simulink model "P2_2"  (R2024b)
settings: Solver=VariableStepAuto  StartTime=0.0  StopTime=0.1  MaxStep=T*samples  RelTol=1e-3
values from neighbouring files (symbols this model uses):
  C = 200e-6    (= 0.0002)    [P2_2Cuestion5.m]
  R = R_vector(i)    [P2_2Cuestion5.m]
  T = 1/f    (= 2.5e-05)    [P2_2Cuestion5.m]
libraries: spsMultimeterLib x4, spsSeriesRLCBranchLib x3, spsMeanLib x3, spsVoltageMeasurementLib x2, spsDiodeLib x1, spsIdealSwitchLib x1, spsRMSLib x1, spsDCVoltageSourceLib x1, sps_lib x1
settings Model: Creator=pablo  LastModifiedBy=Pablo
settings DataIOCC: ReturnWorkspaceOutputs=off

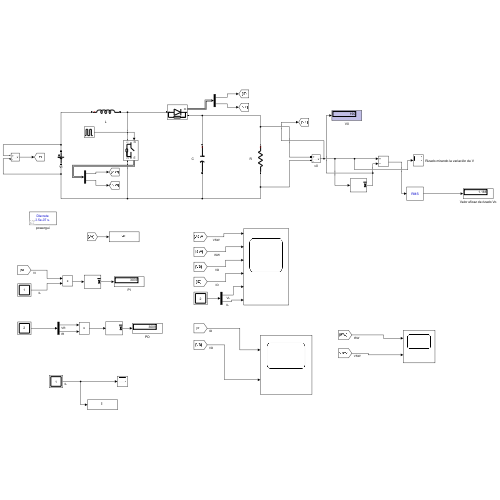
[thumbnail: Simulink's stored preview of the top-level diagram]
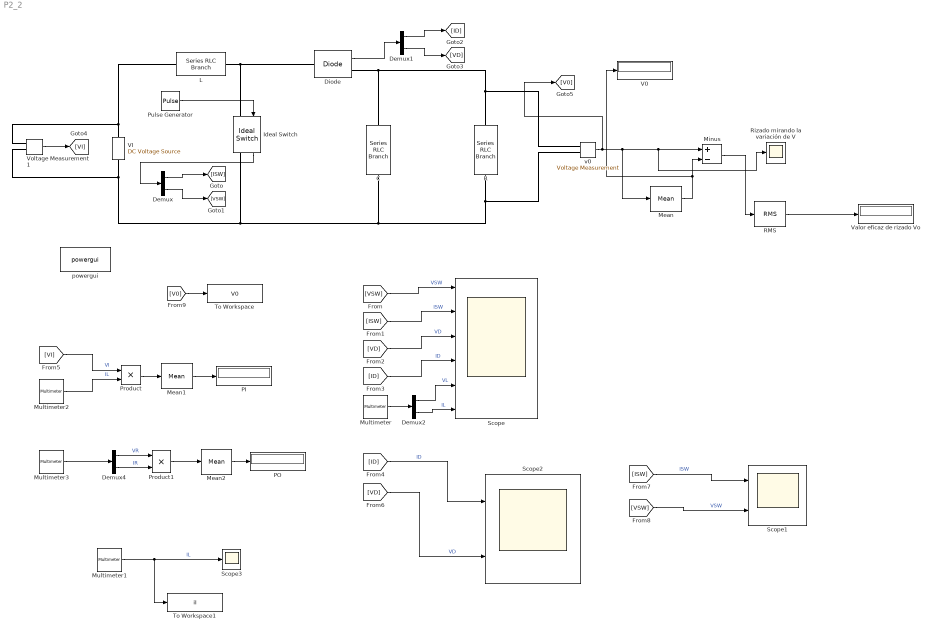
== system P2_2 ==
  C : spsSeriesRLCBranchLib/Series RLC Branch  LConnTagsString=__new0  RConnTagsString=__new0  BranchType=C  Resistance=1  Inductance=1e-3  SetiL0=off  InitialCurrent=0  Capacitance=C  Setx0=off  InitialVoltage=0  Measurements=Branch voltage and current
  Demux{,1..2,4} (4 alike) : Demux  Outputs=2
  Diode : spsDiodeLib/Diode  Ron=0.001  Lon=0  Vf=0.8  IC=0  UseSnubber=0  Rs=500  Cs=250e-9  Measurements=on
  Ideal Switch : spsIdealSwitchLib/Ideal Switch  Ron=0.001  Lon=0  IC=0  Rs=1e5  Cs=inf  Measurements=on
  L : spsSeriesRLCBranchLib/Series RLC Branch  LConnTagsString=__new0  RConnTagsString=__new0  BranchType=L  Resistance=1  Inductance=1e-5  SetiL0=off  InitialCurrent=0  Capacitance=1e-6  Setx0=off  InitialVoltage=0  Measurements=Branch voltage and current
  Mean : spsMeanLib/Mean  Freq=f  Vinit=0  Ts=0
  Mean1 : spsMeanLib/Mean  Freq=f  Vinit=0  Ts=0
  Mean2 : spsMeanLib/Mean  Freq=f  Vinit=0  Ts=0
  Minus : Sum  Inputs=+-
  Multimeter : spsMultimeterLib/Multimeter  L=7  sel=[2 6]  yselected={}  Gain=[1 1]  OutputType=Complex  PlotAtSimulationStop=off  PhasorSimulation=off
  Multimeter1 : spsMultimeterLib/Multimeter  L=7  sel=6  yselected={}  Gain=1  OutputType=Complex  PlotAtSimulationStop=off  PhasorSimulation=off
  Multimeter2 : spsMultimeterLib/Multimeter  L=7  sel=6  yselected={}  Gain=1  OutputType=Complex  PlotAtSimulationStop=off  PhasorSimulation=off
  Multimeter3 : spsMultimeterLib/Multimeter  L=7  sel=[3 7]  yselected={}  Gain=[1 1]  OutputType=Complex  PlotAtSimulationStop=off  PhasorSimulation=off
  PI : Display
  PO : Display
  Product : Product
  Product1 : Product
  Pulse Generator : DiscretePulseGenerator  PulseType=Time based  Period=T  PulseWidth=0.47*100
  R : spsSeriesRLCBranchLib/Series RLC Branch  LConnTagsString=__new0  RConnTagsString=__new0  BranchType=R  Resistance=R  Inductance=1e-3  SetiL0=off  InitialCurrent=0  Capacitance=1e-6  Setx0=off  InitialVoltage=0  Measurements=Branch voltage and current
  RMS : spsRMSLib/RMS  TrueRMS=on  Freq=f  RMSInit=120  Ts=0
  Rizado mirando la variación de V : Scope
  Scope : Scope  NumInputPorts=6
  Scope1 : Scope  NumInputPorts=2
  Scope2 : Scope  NumInputPorts=2
  Scope3 : Scope
  To Workspace : ToWorkspace  VariableName=V0  SaveFormat=Structure With Time  SampleTime=-1
  To Workspace1 : ToWorkspace  VariableName=iI  SaveFormat=Structure With Time  SampleTime=-1
  V0 : Display
  VI : spsDCVoltageSourceLib/DC Voltage Source  Amplitude=80  Measurements=Voltage
  Valor eficaz de rizado Vo : Display
  Voltage Measurement1 : spsVoltageMeasurementLib/Voltage Measurement  PhasorSimulation=off  OutputType=Complex  PSBequivalent=0
  powergui : sps_lib/powergui  Priority=1  SimulationMode=Discrete  SampleTime=2.5e-7  frequency=60  Iterations=50  frequencyindice=0  Pbase=100e6  ErrMax=1e-4  UnitsV=kV  UnitsW=MW  buscounter=0  FunctionMessages=off  echomessages=off  EnableUseOfTLC=off  CurrentSourceSwitches=off  DisableSnubberDevices=off  DisableRonSwitches=off  DisableVfSwitches=off  DisplayEquations=off  AutomaticDiscreteSolvers=off  SolverType=Tustin/Backward Euler (TBE)  Interpol=off  ExternalGateDelay=off  methode=off  Ts=100  x0status=blocks  SPID=on  SwTol=0  HookPort=off  NonlinearTolerance=1e-4  nMaxIteration=100  ContinueOnMaxIteration=off  RestoreLinks=warning  ResistiveCurrentMeasurement=off  Frange=[0:2:500]  Ylog=off  Xlog=on  ShowGrid=off  save=off  variable=ZData  structure=0  ZoomFFT=off  StartTime=0.0  cycles=1  DisplayStyle=1  fundamental=60  FreqAxis=off  MaxFrequency=1000  frequencyindicesteady=1  RmsSteady=1  display=off
  v0 : spsVoltageMeasurementLib/Voltage Measurement  PhasorSimulation=off  OutputType=Complex  PSBequivalent=0
  wires:
  Demux/1 -> [ISW]
  Demux/2 -> [VSW]
  Diode/1 -> Demux1/1
  Demux1/2 -> [VD]
  Demux1/1 -> [ID]
  [VSW] -> Scope/1  "VSW"
  [ISW] -> Scope/2  "ISW"
  [VD] -> Scope/3  "VD"
  [ID] -> Scope/4  "ID"
  Multimeter/1 -> Demux2/1
  Demux2/1 -> Scope/5  "VL"
  Demux2/2 -> Scope/6  "IL"
  v0/1 -> Mean/1, Rizado mirando la variación de V/1, Minus/1, [V0]
  Mean/1 -> V0/1, Minus/2
  Minus/1 -> RMS/1
  Ideal Switch/1 -> Demux/1
  Pulse Generator/1 -> Ideal Switch/1
  [ID] -> Scope2/1  "ID"
  Voltage Measurement1/1 -> [VI]
  [VI] -> Product/1  "VI"
  Multimeter2/1 -> Product/2  "IL"
  Multimeter3/1 -> Demux4/1
  Demux4/1 -> Product1/1  "VR"
  Demux4/2 -> Product1/2  "IR"
  Product/1 -> Mean1/1
  Mean1/1 -> PI/1
  Product1/1 -> Mean2/1
  Mean2/1 -> PO/1
  [VD] -> Scope2/2  "VD"
  [V0] -> To Workspace/1
  [ISW] -> Scope1/1  "ISW"
  [VSW] -> Scope1/2  "VSW"
  Multimeter1/1 -> To Workspace1/1, Scope3/1  "IL"
  RMS/1 -> Valor eficaz de rizado Vo/1
  connections:
  VI/RConn1 -- L/LConn1 -- Voltage Measurement1/LConn1
  Diode/LConn1 -- Ideal Switch/LConn1 -- L/RConn1
  Diode/RConn1 -- v0/LConn1 -- R/LConn1 -- C/LConn1
  C/RConn1 -- Ideal Switch/RConn1 -- Voltage Measurement1/LConn2 -- VI/LConn1 -- R/RConn1 -- v0/LConn2
